simulink model "ff_blackhawk_3dof"  (Simulink 7.0)
settings: Solver=ode45  StartTime=0.0  StopTime=100  RelTol=1e-3
values from neighbouring files (symbols this model uses):
  a = 10*wd    [HelicopterHoverExample.m]
  Int_Sample_Time = 1/1000    (= 0.001)    [HelicopterHoverExample.m]
  Kden = [A1 A0]    [HelicopterHoverExample.m]
  Knum = [B1 B0]    [HelicopterHoverExample.m]
  w_GG = 100 * (2*pi)    (= 628.318530718)    [HelicopterHoverExample.m]
  z_GG = 1/sqrt(2)    [HelicopterHoverExample.m]
undefined symbols (not defined in the file or in its folder): DiscIntNeverNeededParam, plant_den, plant_num
libraries: simulink x2
settings Model: Creator=gabe  LastModifiedBy=gabe

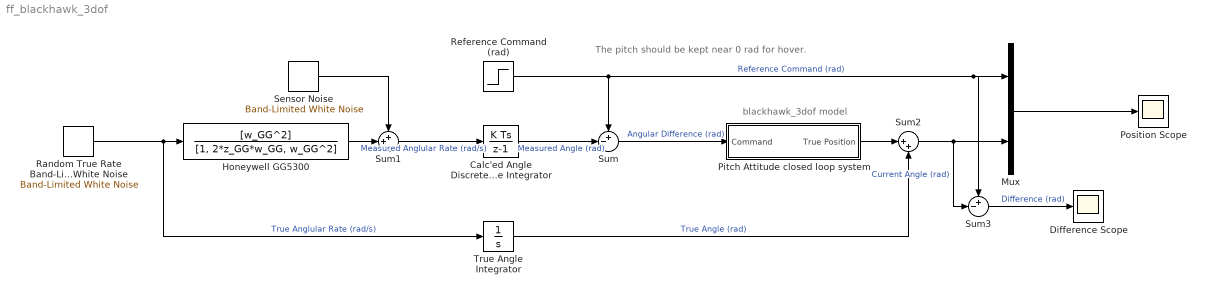
== system ff_blackhawk_3dof ==
  note: The pitch should be kept near 0 rad for hover.
  note: blackhawk_3dof model
  Calc'ed Angle Discrete-Time Integrator : DiscreteIntegrator  SampleTime=Int_Sample_Time  OutDataType=sfix(16)  OutScaling=2^0  ICPrevOutput=DiscIntNeverNeededParam  ICPrevScaledInput=DiscIntNeverNeededParam
  Difference Scope : Scope
      settings: TimeRange=100  YMin=-0.0025  YMax=0.035  SaveName=ff_Err  SampleInput=on  SampleTime=1/1000
  Honeywell GG5300 : TransferFcn  Numerator=[w_GG^2]  Denominator=[1, 2*z_GG*w_GG, w_GG^2]
  Mux : Mux  Inputs=2
  Pitch Attitude closed loop system : Subsystem
  Position Scope : Scope
      settings: TimeRange=100  YMin=0.0955  YMax=0.107  SaveName=ff_Pitch  SampleInput=on  SampleTime=1/1000
  Random True Rate Band-Limited White Noise : simulink/Sources/Band-Limited White Noise  SystemSampleTime=-1  Cov=1E-5  Ts=0.1  seed=ff_blackhawk_rate_seed
  Reference Command (rad) : Step  Time=10  After=0.1  SampleTime=0
  Sensor Noise : simulink/Sources/Band-Limited White Noise  SystemSampleTime=-1  Cov=1E-10  Ts=1/10000  seed=ff_blackhawk_sensor_seed
  Sum : Sum  Inputs=+-|  OutDataType=sfix(16)  OutScaling=2^0
  Sum1 : Sum  Inputs=++|  OutDataType=sfix(16)  OutScaling=2^0
  Sum2 : Sum  Inputs=|++  OutDataType=sfix(16)  OutScaling=2^0
  Sum3 : Sum  Inputs=+-|  OutDataType=sfix(16)  OutScaling=2^0
  True Angle Integrator : Integrator
  wires:
  Mux/1 -> Position Scope/1
  Pitch Attitude closed loop system/1(True Position) -> Sum2/1
  Reference Command (rad)/1 -> Sum/1, Mux/1, Sum3/1  "Reference Command (rad)"
  Calc'ed Angle Discrete-Time Integrator/1 -> Sum/2  "Measured Angle (rad)"
  Sum/1 -> Pitch Attitude closed loop system/1(Command)  "Angular Difference (rad)"
  Random True Rate Band-Limited White Noise/1 -> Honeywell GG5300/1, True Angle Integrator/1  "True Anglular Rate (rad/s)"
  Sum1/1 -> Calc'ed Angle Discrete-Time Integrator/1  "Measured Anglular Rate (rad/s)"
  Sensor Noise/1 -> Sum1/1
  True Angle Integrator/1 -> Sum2/2  "True Angle (rad)"
  Sum2/1 -> Mux/2, Sum3/2  "Current Angle (rad)"
  Honeywell GG5300/1 -> Sum1/2
  Sum3/1 -> Difference Scope/1  "Difference (rad)"

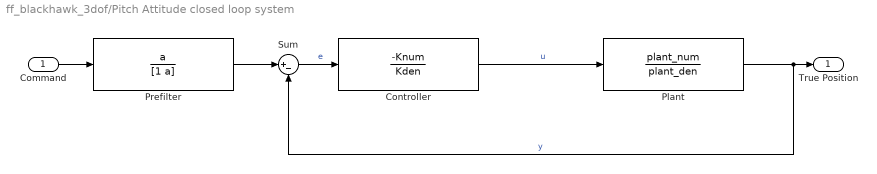
== system ff_blackhawk_3dof/Pitch Attitude closed loop system ==
  Command : Inport
  Controller : TransferFcn  Numerator=-Knum  Denominator=Kden
  Plant : TransferFcn  Numerator=plant_num  Denominator=plant_den
  Prefilter : TransferFcn  Numerator=a  Denominator=[1 a]
  Sum : Sum  Inputs=|+-  OutDataType=sfix(16)  OutScaling=2^0
  True Position : Outport
  wires:
  Plant/1 -> Sum/2, True Position/1  "y"
  Controller/1 -> Plant/1  "u"
  Sum/1 -> Controller/1  "e"
  Prefilter/1 -> Sum/1
  Command/1 -> Prefilter/1
